simulink model "sfcndemo_dtype_io"  (Simulink 7.6)
settings: Solver=FixedStepDiscrete  StartTime=0.0  StopTime=10.0  RelTol=1e-3
Description:
  | Data-Typed I/O Using a C-MEX S-function
settings Model: Creator=The MathWorks Inc.  ExtModeAutoUpdateStatusClock=off
settings OptimizationCC: BlockReduction=off  BooleanDataType=off  InitFltsAndDblsToZero=on
settings DebuggingCC: SaveWithParameterizedLinksMsg=none  SignalResolutionControl=TryResolveAllWithWarning  SolverPrmCheckMsg=none  MultiTaskDSMMsg=warning  MultiTaskCondExecSysMsg=none
settings HardwareCC: TargetUnknown=on
settings RTWCC: IncludeERTFirstTime=on
settings CodeAppCC: CustomSymbolStrFcn=$F$N$M
settings GRTTargetCC: TargetFcnLib=ansi_tfl_tmw.mat

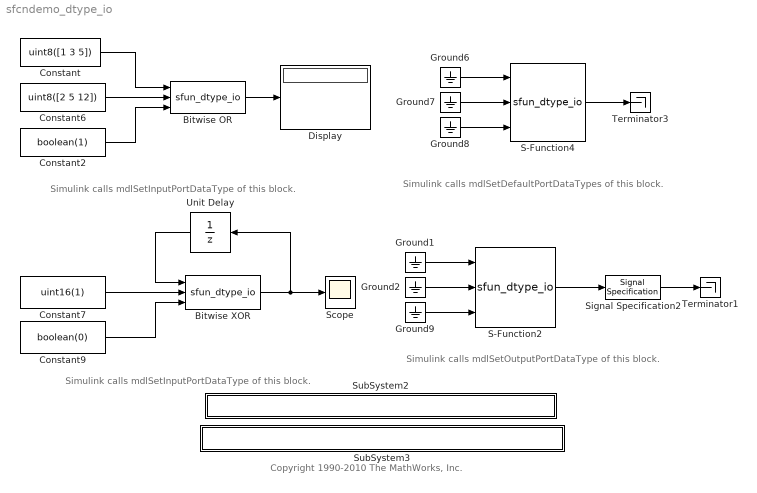
== system sfcndemo_dtype_io ==
  note: Simulink calls mdlSetDefaultPortDataTypes of this block.
  note: Simulink calls mdlSetOutputPortDataType of this block.
  note: Simulink calls mdlSetInputPortDataType of this block.
  note: Simulink calls mdlSetInputPortDataType of this block.
  note: Copyright 1990-2010 The MathWorks, Inc.
  Bitwise OR : S-Function  FunctionName=sfun_dtype_io  EnableBusSupport=off
  Bitwise XOR : S-Function  FunctionName=sfun_dtype_io  EnableBusSupport=off
  Constant : Constant  Value=uint8([1 3 5])
  Constant2 : Constant  Value=boolean(1)
  Constant6 : Constant  Value=uint8([2 5 12])
  Constant7 : Constant  Value=uint16(1)
  Constant9 : Constant  Value=boolean(0)
  Display : Display
  Ground{1..2,6..9} (6 alike) : Ground
  S-Function2 : S-Function  FunctionName=sfun_dtype_io  EnableBusSupport=off
  S-Function4 : S-Function  FunctionName=sfun_dtype_io  EnableBusSupport=off
  Scope : Scope
      settings: TimeRange=10  YMin=-0.5  YMax=1.5
  Signal Specification2 : SignalSpecification  OutDataTypeStr=uint32
  SubSystem2 : Subsystem  mask{filename=sfun_dtype_io.c}
      mask init:
      | x=sfundemo_maskdisp;
      settings: AttributesFormatString=\n  OpenFcn=sfundemo_openfcn
      mask Display: disp(x);
  SubSystem3 : Subsystem  mask{filename=sfun_dtype_io.tlc}
      mask init:
      | x=sfundemo_maskdisp;
      settings: AttributesFormatString=\n  OpenFcn=sfundemo_openfcn
      mask Display: disp(x);
  Terminator1 : Terminator
  Terminator3 : Terminator
  Unit Delay : UnitDelay
  wires:
  Constant/1 -> Bitwise OR/1
  Bitwise OR/1 -> Display/1
  Constant2/1 -> Bitwise OR/3
  Constant6/1 -> Bitwise OR/2
  Bitwise XOR/1 -> Unit Delay/1, Scope/1
  Constant9/1 -> Bitwise XOR/3
  Constant7/1 -> Bitwise XOR/2
  Unit Delay/1 -> Bitwise XOR/1
  Ground6/1 -> S-Function4/1
  S-Function4/1 -> Terminator3/1
  Ground7/1 -> S-Function4/2
  Ground8/1 -> S-Function4/3
  Ground1/1 -> S-Function2/1
  S-Function2/1 -> Signal Specification2/1
  Ground2/1 -> S-Function2/2
  Ground9/1 -> S-Function2/3
  Signal Specification2/1 -> Terminator1/1

== system sfcndemo_dtype_io/SubSystem2 ==

== system sfcndemo_dtype_io/SubSystem3 ==
